simulink model "PasiveBalancerCopy"  (R2021a)
settings: Solver=VariableStepAuto  StartTime=0.0  StopTime=600  RelTol=1e-3
undefined symbols (not defined in the file): Ion, Lithium
libraries: spsSeriesRLCBranchLib x8, spsBatteryLib x6, spsIGBTLib x6, spsIdealSwitchLib x4, spsDCVoltageSourceLib x2, spspowerguiLib x1
settings Model: Creator=jafar  LastModifiedBy=jafar

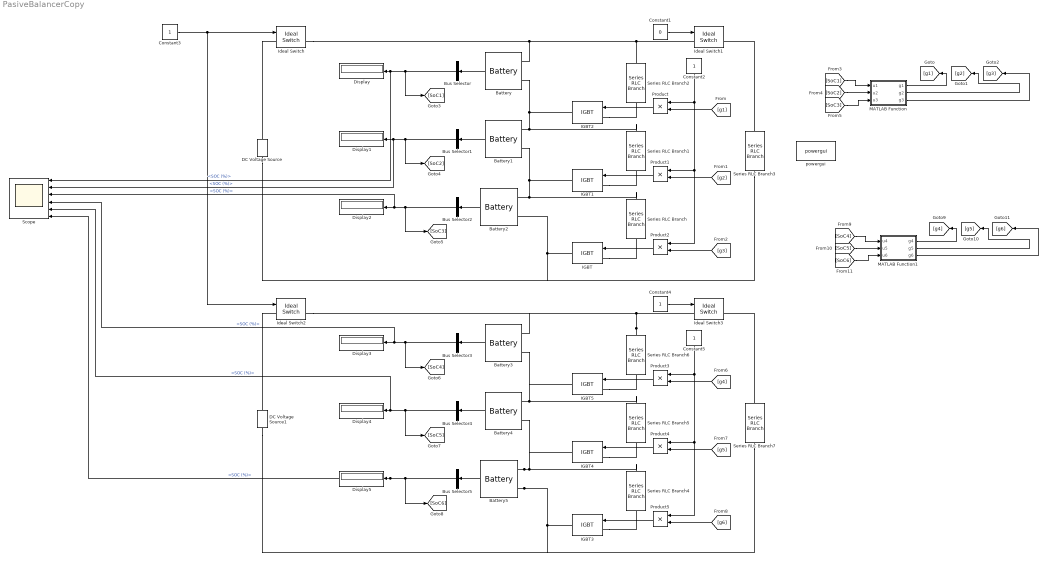
== system PasiveBalancerCopy ==
  Battery : spsBatteryLib/Battery  BatType=Lithium-Ion  ShowTempParam=off  ThermalPreset=no  ShowAgeParam=off  NomV=3.7  NomQ=5.4  SOC=20  Batt_Tr=30  PresetModel=on  MaxQ=5.4  MinV=2.775  FullV=4.3068  Dis_rate=2.3478  R=0.0068519  Normal_OP=4.8835  expZone="[3.9974      0.2653]"  current=[6.5 13 32.5]  Units=Time  Tci=20  NomT=20  T2=-30  MaxQ2=4.8  FullV2=7.1  Normal_OP2=5.655  expZone2="[6.58           1]"  Rca=0.6  ti=2000  Dp=0  Neq0=0  Tsim=1e6  Ta1=25  Qeol=5.4*0.9  Reol=0.013333*1.2  Char_age=[2.3478, 3]  Dis_age=[2.3478, 10]  N1=1500  N2=10500  N3=1000  N4=1400  Ta2=45  N5=950
  Battery1 : spsBatteryLib/Battery  BatType=Lithium-Ion  ShowTempParam=off  ThermalPreset=no  ShowAgeParam=off  NomV=3.7  NomQ=5.4  SOC=25  Batt_Tr=30  PresetModel=on  MaxQ=5.4  MinV=2.775  FullV=4.3068  Dis_rate=2.3478  R=0.0068519  Normal_OP=4.8835  expZone="[3.9974      0.2653]"  current=[6.5 13 32.5]  Units=Time  Tci=20  NomT=20  T2=-30  MaxQ2=4.8  FullV2=7.1  Normal_OP2=5.655  expZone2="[6.58           1]"  Rca=0.6  ti=2000  Dp=0  Neq0=0  Tsim=1e6  Ta1=25  Qeol=5.4*0.9  Reol=0.013333*1.2  Char_age=[2.3478, 3]  Dis_age=[2.3478, 10]  N1=1500  N2=10500  N3=1000  N4=1400  Ta2=45  N5=950
  Battery2 : spsBatteryLib/Battery  BatType=Lithium-Ion  ShowTempParam=off  ThermalPreset=no  ShowAgeParam=off  NomV=3.7  NomQ=5.4  SOC=28  Batt_Tr=30  PresetModel=on  MaxQ=5.4  MinV=2.775  FullV=4.3068  Dis_rate=2.3478  R=0.0068519  Normal_OP=4.8835  expZone="[3.9974      0.2653]"  current=[6.5 13 32.5]  Units=Time  Tci=20  NomT=20  T2=-30  MaxQ2=4.8  FullV2=7.1  Normal_OP2=5.655  expZone2="[6.58           1]"  Rca=0.6  ti=2000  Dp=0  Neq0=0  Tsim=1e6  Ta1=25  Qeol=5.4*0.9  Reol=0.013333*1.2  Char_age=[2.3478, 3]  Dis_age=[2.3478, 10]  N1=1500  N2=10500  N3=1000  N4=1400  Ta2=45  N5=950
  Battery3 : spsBatteryLib/Battery  BatType=Lithium-Ion  ShowTempParam=off  ThermalPreset=no  ShowAgeParam=off  NomV=3.7  NomQ=5.4  SOC=30  Batt_Tr=30  PresetModel=on  MaxQ=5.4  MinV=2.775  FullV=4.3068  Dis_rate=2.3478  R=0.0068519  Normal_OP=4.8835  expZone="[3.9974      0.2653]"  current=[6.5 13 32.5]  Units=Time  Tci=20  NomT=20  T2=-30  MaxQ2=4.8  FullV2=7.1  Normal_OP2=5.655  expZone2="[6.58           1]"  Rca=0.6  ti=2000  Dp=0  Neq0=0  Tsim=1e6  Ta1=25  Qeol=5.4*0.9  Reol=0.013333*1.2  Char_age=[2.3478, 3]  Dis_age=[2.3478, 10]  N1=1500  N2=10500  N3=1000  N4=1400  Ta2=45  N5=950
  Battery4 : spsBatteryLib/Battery  BatType=Lithium-Ion  ShowTempParam=off  ThermalPreset=no  ShowAgeParam=off  NomV=3.7  NomQ=5.4  SOC=35  Batt_Tr=30  PresetModel=on  MaxQ=5.4  MinV=2.775  FullV=4.3068  Dis_rate=2.3478  R=0.0068519  Normal_OP=4.8835  expZone="[3.9974      0.2653]"  current=[6.5 13 32.5]  Units=Time  Tci=20  NomT=20  T2=-30  MaxQ2=4.8  FullV2=7.1  Normal_OP2=5.655  expZone2="[6.58           1]"  Rca=0.6  ti=2000  Dp=0  Neq0=0  Tsim=1e6  Ta1=25  Qeol=5.4*0.9  Reol=0.013333*1.2  Char_age=[2.3478, 3]  Dis_age=[2.3478, 10]  N1=1500  N2=10500  N3=1000  N4=1400  Ta2=45  N5=950
  Battery5 : spsBatteryLib/Battery  BatType=Lithium-Ion  ShowTempParam=off  ThermalPreset=no  ShowAgeParam=off  NomV=3.7  NomQ=5.4  SOC=50  Batt_Tr=30  PresetModel=on  MaxQ=5.4  MinV=2.775  FullV=4.3068  Dis_rate=2.3478  R=0.0068519  Normal_OP=4.8835  expZone="[3.9974      0.2653]"  current=[6.5 13 32.5]  Units=Time  Tci=20  NomT=20  T2=-30  MaxQ2=4.8  FullV2=7.1  Normal_OP2=5.655  expZone2="[6.58           1]"  Rca=0.6  ti=2000  Dp=0  Neq0=0  Tsim=1e6  Ta1=25  Qeol=5.4*0.9  Reol=0.013333*1.2  Char_age=[2.3478, 3]  Dis_age=[2.3478, 10]  N1=1500  N2=10500  N3=1000  N4=1400  Ta2=45  N5=950
  Bus Selector{,1..5} (6 alike) : BusSelector  OutputSignals=SOC (%)
  Constant1 : Constant  Value=0
  Constant{2..5} (4 alike) : Constant
  DC Voltage Source : spsDCVoltageSourceLib/DC Voltage Source  Amplitude=12  Measurements=None
  DC Voltage Source1 : spsDCVoltageSourceLib/DC Voltage Source  Amplitude=12  Measurements=None
  Display{,1..5} (6 alike) : Display
  IGBT{,1..5} (6 alike) : spsIGBTLib/IGBT  Ron=0.001  Lon=0  Vf=1  Tf=1e-6  Tt=2e-6  IC=0  Rs=1e5  Cs=inf  Measurements=off
  Ideal Switch{,1..3} (4 alike) : spsIdealSwitchLib/Ideal Switch  Ron=0.001  Lon=0  IC=0  Rs=1e5  Cs=inf  Measurements=on
  MATLAB Function : MATLAB Function  TreatAsAtomicUnit=on
  MATLAB Function1 : MATLAB Function  TreatAsAtomicUnit=on
  Product{,1..5} (6 alike) : Product
  Scope : Scope  NumInputPorts=6
  Series RLC Branch{,1..7} (8 alike) : spsSeriesRLCBranchLib/Series RLC Branch  LConnTagsString=__new0  RConnTagsString=__new0  BranchType=R  Resistance=1  Inductance=1e-3  SetiL0=off  InitialCurrent=0  Capacitance=1e-6  Setx0=off  InitialVoltage=0  Measurements=None
  powergui : spspowerguiLib/powergui  Priority=1  SimulationMode=Continuous  SampleTime=50e-6  frequency=60  Iterations=50  frequencyindice=0  Pbase=100e6  ErrMax=1e-4  UnitsV=kV  UnitsW=MW  buscounter=0  FunctionMessages=off  echomessages=off  EnableUseOfTLC=off  CurrentSourceSwitches=off  DisableSnubberDevices=off  DisableRonSwitches=off  DisableVfSwitches=off  DisplayEquations=off  AutomaticDiscreteSolvers=off  SolverType=Tustin/Backward Euler (TBE)  Interpol=off  ExternalGateDelay=off  methode=off  Ts=100  x0status=blocks  SPID=on  SwTol=0  HookPort=off  NonlinearTolerance=1e-4  nMaxIteration=100  ContinueOnMaxIteration=off  RestoreLinks=warning  ResistiveCurrentMeasurement=off  Frange=[0:2:500]  Ylog=off  Xlog=on  ShowGrid=off  save=off  variable=ZData  structure=0  ZoomFFT=off  StartTime=0.0  cycles=1  DisplayStyle=1  fundamental=60  FreqAxis=off  MaxFrequency=1000  frequencyindicesteady=1  RmsSteady=1  display=off
  wires:
  Constant3/1 -> Ideal Switch/1, Ideal Switch2/1
  Constant1/1 -> Ideal Switch1/1
  Battery/1 -> Bus Selector/1
  Battery1/1 -> Bus Selector1/1
  Battery2/1 -> Bus Selector2/1
  Bus Selector/1 -> [SoC1], Scope/1, Display/1  "<SOC (%)>"
  Bus Selector1/1 -> [SoC2], Scope/2, Display1/1  "<SOC (%)>"
  Bus Selector2/1 -> [SoC3], Scope/3, Display2/1  "<SOC (%)>"
  Product/1 -> IGBT2/1
  Product1/1 -> IGBT1/1
  Product2/1 -> IGBT/1
  Constant2/1 -> Product/1, Product1/1, Product2/1
  [g1] -> Product/2
  [g2] -> Product1/2
  [g3] -> Product2/2
  MATLAB Function/1(g1) -> [g1]
  MATLAB Function/2(g2) -> [g2]
  MATLAB Function/3(g3) -> [g3]
  [SoC1] -> MATLAB Function/1(u1)
  [SoC2] -> MATLAB Function/2(u2)
  [SoC3] -> MATLAB Function/3(u3)
  Constant5/1 -> Product3/1, Product4/1, Product5/1
  Battery5/1 -> Bus Selector5/1
  [g6] -> Product5/2
  Bus Selector5/1 -> [SoC6], Scope/6, Display5/1  "<SOC (%)>"
  Product4/1 -> IGBT4/1
  Bus Selector3/1 -> [SoC4], Scope/4, Display3/1  "<SOC (%)>"
  [g4] -> Product3/2
  Bus Selector4/1 -> [SoC5], Scope/5, Display4/1  "<SOC (%)>"
  Constant4/1 -> Ideal Switch3/1
  Product5/1 -> IGBT3/1
  Battery3/1 -> Bus Selector3/1
  Product3/1 -> IGBT5/1
  [g5] -> Product4/2
  Battery4/1 -> Bus Selector4/1
  [SoC6] -> MATLAB Function1/3(u6)
  [SoC4] -> MATLAB Function1/1(u4)
  MATLAB Function1/1(g4) -> [g4]
  MATLAB Function1/3(g6) -> [g6]
  MATLAB Function1/2(g5) -> [g5]
  [SoC5] -> MATLAB Function1/2(u5)
  connections:
  Battery/LConn2 -- IGBT2/RConn1 -- Series RLC Branch1/LConn1 -- Battery1/LConn1
  Battery1/LConn2 -- IGBT1/RConn1 -- Series RLC Branch/LConn1 -- Battery2/LConn1
  IGBT/RConn1 -- DC Voltage Source/LConn1 -- Series RLC Branch3/RConn1 -- Battery2/LConn2
  IGBT/LConn1 -- Series RLC Branch/RConn1
  IGBT1/LConn1 -- Series RLC Branch1/RConn1
  IGBT2/LConn1 -- Series RLC Branch2/RConn1
  Battery/LConn1 -- Ideal Switch/RConn1 -- Ideal Switch1/LConn1 -- Series RLC Branch2/LConn1
  Ideal Switch/LConn1 -- DC Voltage Source/RConn1
  Series RLC Branch3/LConn1 -- Ideal Switch1/RConn1
  Series RLC Branch6/LConn1 -- Ideal Switch3/LConn1 -- Battery3/LConn1 -- Ideal Switch2/RConn1
  Battery4/LConn1 -- Battery3/LConn2 -- IGBT5/RConn1 -- Series RLC Branch5/LConn1
  Battery5/LConn2 -- IGBT3/RConn1 -- DC Voltage Source1/LConn1 -- Series RLC Branch7/RConn1
  Battery5/LConn1 -- Series RLC Branch4/LConn1 -- Battery4/LConn2 -- IGBT4/RConn1
  IGBT5/LConn1 -- Series RLC Branch6/RConn1
  Series RLC Branch7/LConn1 -- Ideal Switch3/RConn1
  IGBT3/LConn1 -- Series RLC Branch4/RConn1
  Ideal Switch2/LConn1 -- DC Voltage Source1/RConn1
  IGBT4/LConn1 -- Series RLC Branch5/RConn1

== matlab function PasiveBalancerCopy/MATLAB Function1 ==
  data: u4 input; g4 output; u5 input; u6 input; g5 output; g6 output
function [g4,g5,g6] = fcn(u4,u5,u6)

u4 = u4*1000;
u5 = u5*1000;
u6 = u6*1000;

u4 = int32(u4);
u5 = int32(u5);
u6 = int32(u6);

if u4>u5||u4>u6
    g4 = 1;
else
    g4 = 0;
end
    
if u5>u4||u5>u6
    g5 = 1;
else
    g5 = 0;
end

if u6>u4||u6>u5
    g6 = 1;
else
    g6 = 0;
end
end

== matlab function PasiveBalancerCopy/MATLAB Function ==
  data: u1 input; g1 output; u2 input; u3 input; g2 output; g3 output
function [g1,g2,g3] = fcn(u1,u2,u3)

u1 = u1*1000;
u2 = u2*1000;
u3 = u3*1000;

u1 = int32(u1);
u2 = int32(u2);
u3 = int32(u3);

if u1>u2||u1>u3
    g1 = 1;
else
    g1 = 0;
end
    
if u2>u1||u2>u3
    g2 = 1;
else
    g2 = 0;
end

if u3>u1||u3>u2
    g3 = 1;
else
    g3 = 0;
end

end
